simulink model "ctrl_student_caseb"  (R2015a)
settings: Solver=ode4  StartTime=0.0  StopTime=inf  FixedStep=0.01  RelTol=1e-3
settings Model: CovSFcnEnable=off  Creator=mclab  LastModifiedBy=MCLab
settings DebuggingCC: SolverPrmCheckMsg=warning  InheritedTsInSrcMsg=none
settings RTWCC: SystemTargetFile=NIVeriStand_VxWorks.tlc  TemplateMakefile=NIVeriStand_VxWorks.tmf  Description=NI VeriStand VxWorks Real-Time Target for Release 2007b or later
settings STFCustomTargetCC: GenerateSampleERTMain=off  GeneratePreprocessorConditionals=Disable all  ERTCustomFileBanners=off  MatFileLogging=on  SupportNonInlinedSFcns=on  SupportVariableSizeSignals=off  MATLABClassNameForMDSCustomization=Simulink.SoftwareTarget.TargetSpecificTriggerConfigurationBase  GRTInterface=on  SystemTargetFile=NIVeriStand_VxWorks.tlc

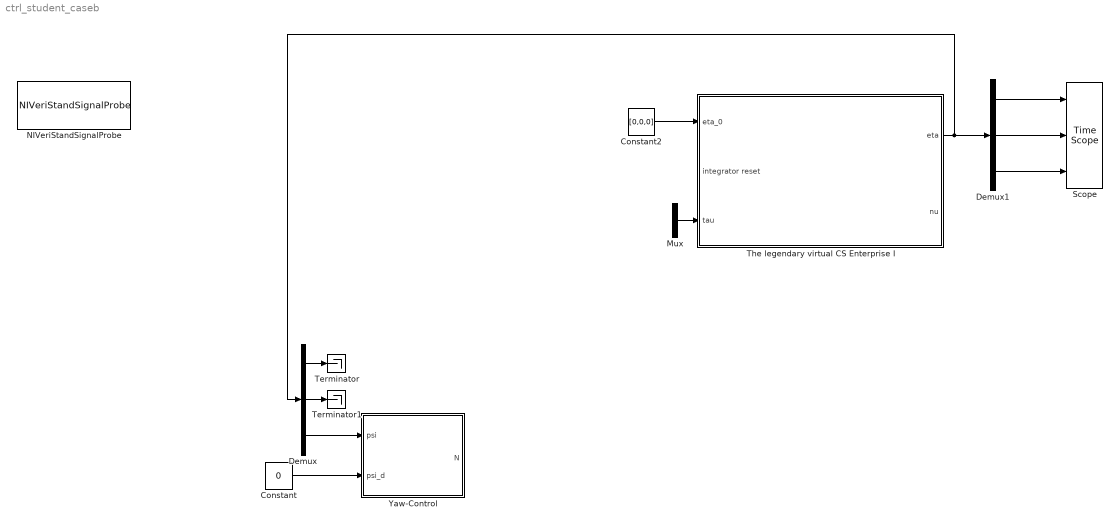
== system ctrl_student_caseb ==
  Constant : Constant  Value=0
  Constant2 : Constant  Value=[0,0,0]
  Demux : Demux  Outputs=3
  Demux1 : Demux  Outputs=3
  Mux : Mux  Inputs=3
  NIVeriStandSignalProbe : S-Function  FunctionName=NIVeriStandSignalProbe  Parameters=1
  Scope : TimeScope  NumInputPorts=3
  Terminator : Terminator
  Terminator1 : Terminator
  The legendary virtual CS Enterprise I : Subsystem
  Yaw-Control : Subsystem
  wires:
  Constant2/1 -> The legendary virtual CS Enterprise I/1(eta_0)
  Mux/1 -> The legendary virtual CS Enterprise I/3(tau)
  The legendary virtual CS Enterprise I/1(eta) -> Demux1/1, Demux/1
  Demux/3 -> Yaw-Control/1(psi)
  Constant/1 -> Yaw-Control/2(psi_d)
  Demux1/2 -> Scope/2
  Demux1/3 -> Scope/3
  Demux1/1 -> Scope/1
  Demux/1 -> Terminator/1
  Demux/2 -> Terminator1/1

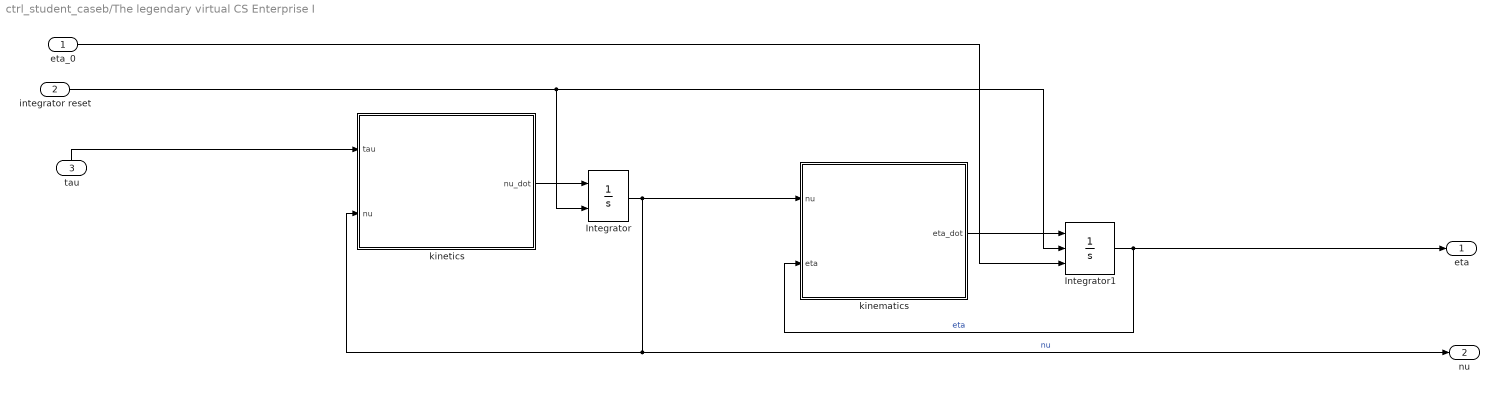
== system ctrl_student_caseb/The legendary virtual CS Enterprise I ==
  eta_0 : Inport
  integrator reset : Inport  Port=2
  tau : Inport  Port=3
  Integrator : Integrator  ExternalReset=rising  InitialCondition=[0 0 0]'
  Integrator1 : Integrator  ExternalReset=rising  InitialConditionSource=external  InitialCondition=[0 0 0]'
  kinematics : MATLAB Function  TreatAsAtomicUnit=on
  kinetics : MATLAB Function  TreatAsAtomicUnit=on
  eta : Outport
  nu : Outport  Port=2
  wires:
  eta_0/1 -> Integrator1/3
  integrator reset/1 -> Integrator1/2, Integrator/2
  Integrator1/1 -> eta/1, kinematics/2(eta)  "eta"
  kinematics/1(eta_dot) -> Integrator1/1
  Integrator/1 -> nu/1, kinetics/2(nu), kinematics/1(nu)  "nu"
  kinetics/1(nu_dot) -> Integrator/1
  tau/1 -> kinetics/1(tau)

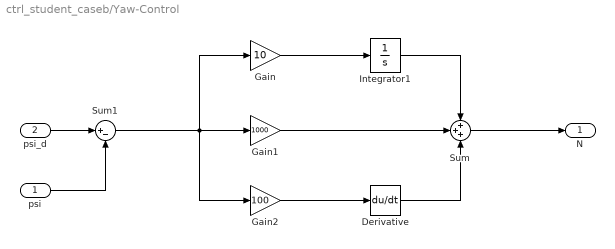
== system ctrl_student_caseb/Yaw-Control ==
  psi : Inport
  psi_d : Inport  Port=2
  Derivative : Derivative
  Gain : Gain  Gain=10
  Gain1 : Gain  Gain=1000
  Gain2 : Gain  Gain=100
  Integrator1 : Integrator
  Sum : Sum  Inputs=+++
  Sum1 : Sum  Inputs=|+-
  N : Outport
  wires:
  psi_d/1 -> Sum1/1
  Sum1/1 -> Gain2/1, Gain/1, Gain1/1
  Gain1/1 -> Sum/2
  Gain/1 -> Integrator1/1
  Sum/1 -> N/1
  Integrator1/1 -> Sum/1
  psi/1 -> Sum1/2
  Gain2/1 -> Derivative/1
  Derivative/1 -> Sum/3

== matlab function ctrl_student_caseb/The legendary virtual CS Enterprise I/kinematics ==
  data: nu input; eta_dot output; eta input
function eta_dot = CSE1_eta_dot(nu,eta)

psi = eta(3);

J = [cos(psi) -sin(psi) 0
     sin(psi) cos(psi)  0
     0        0         1];

eta_dot = J*nu;

== matlab function ctrl_student_caseb/The legendary virtual CS Enterprise I/kinetics ==
  data: tau input; nu_dot output; nu input
function nu_dot = CSE1_nu_dot(tau,nu)

u   = nu(1);
v   = nu(2);
r   = nu(3);

tau = [tau(1);tau(2);tau(3)];
%% MATRICES

m    = 14.79;   I_z  =  1.7600;   x_g = 0.0375;       % x_g  =  0.0460; % Table B.1


%% Added mass
X_ud  =     -2.0;											% Table B.1
					Y_vd =     -10.0;	N_vd =    -0.0;		% Table B.1
					Y_rd =      -0.0;	N_rd =    -1.0;		% Table B.1

%% Total mass matrix
m_11 = m-X_ud;
m_22 = m-Y_vd;
m_23 = m*x_g-Y_rd;
m_32 = m*x_g-N_vd;
m_33 = I_z-N_rd;

M    = [m_11 0    0
        0    m_22 m_23
        0    m_32 m_33];
	
%% Damping coefficients
% Comments at the end of the lines indicate the old values used.
X_u		= -0.6555;		X_v		= 0;
X_uu 	= 0.3545;		X_vv	= -2.443;
X_uuu 	= -3.787;		X_vvv	= 0;

						Y_v		= -1.33; 			Y_r		= -7.250; % Y_r
						Y_vv	= -2.776;			Y_rr	= -3.450; % Y_rr
						Y_vvv	= -64.91;			Y_rrr	= 0;
						
						Y_rv	= -0.805;			Y_vr	= -0.845; % Y_rv, Y_vr

						N_v		= 0;				N_r		= -1.900; % N_r
						N_vv	= -0.2088;			N_rr	= -0.750; % N_rr
						N_vvv	= 0;				N_rrr	= 0;
						
						N_rv	= 0.130;			N_vr	= 0.080; % N_rv, N_vr

%% Correolis matrix
c_13 = -(m-Y_vd)*v-(m*x_g-Y_rd)*r;
c_23 = (m-X_ud)*u;
C    = [0     0     c_13
        0     0     c_23
        -c_13 -c_23 0   ];

%% Assembly of the damping matrix
d_11 = -X_u - X_uu*u - X_uuu*u^2;
d_22 = -Y_v - Y_vv*v - Y_vvv*v^2 - Y_rv*abs(r);
d_33 = -N_r - N_rr*abs(r) - N_rrr*r^2 - N_vr*abs(v); % using abs(r)

d_12 = -X_v - X_vv*v - X_vvv*v^2;
d_23 = -Y_r - Y_rr*abs(r) - Y_rrr*r^2 - Y_vr*abs(v);
d_32 = -N_v - N_vv*v - N_vvv*v^2 - N_rv*abs(r);

D    = [d_11 d_12 0
        0    d_22 d_23
        0    d_32 d_33];



%% CALCULATION
nu_dot = M\(tau-(C+D)*nu);
